simulink model "sampleModel1690_2_sub"  (R2023a)
settings: Solver=VariableStepAuto  StartTime=0.0  StopTime=10.0  RelTol=1e-3
libraries: hdlsllib x1, simulink x1
settings Model: Creator=user1  LastModifiedBy=user1

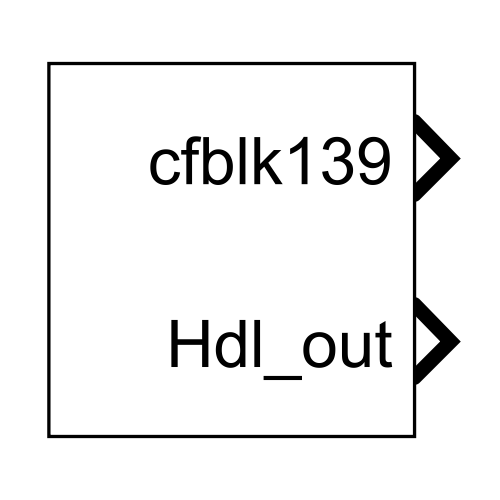
[thumbnail: Simulink's stored preview of the top-level diagram]
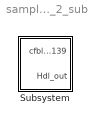
== system sampleModel1690_2_sub ==
  Subsystem : Subsystem

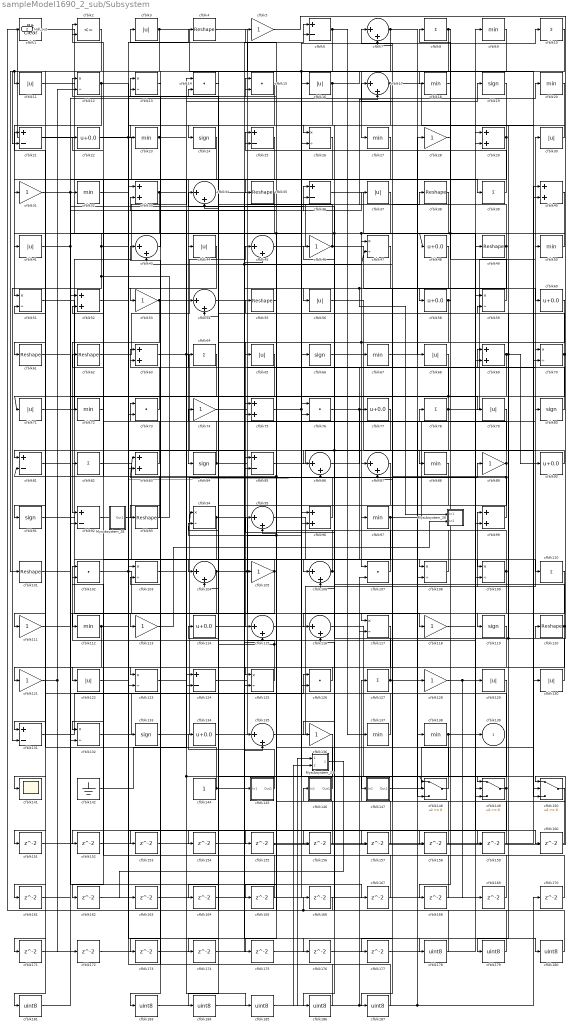
== system sampleModel1690_2_sub/Subsystem ==
  Mysubsystem_23 : Subsystem  TreatAsAtomicUnit=on  RTWFcnName=Mysubsystem_23
      settings: RTWFcnNameOpts=User specified  RTWFileNameOpts=Use function name
  Mysubsystem_26 : Subsystem  TreatAsAtomicUnit=on  RTWFcnName=Mysubsystem_26
      settings: RTWFcnNameOpts=User specified  RTWFileNameOpts=Use function name
  Mysubsystem_28 : Subsystem  TreatAsAtomicUnit=on  RTWFcnName=Mysubsystem_28
      settings: RTWFcnNameOpts=User specified  RTWFileNameOpts=Use function name
  cfblk1 : simulink/Logic and Bit Operations/Bit Clear  iBit=0
      settings: LibrarySourceBlock=|
      | hdlsllib/Logic and Bit
      | Operations/Bit Clear
  cfblk{8,10,39,64,78,82,110,127} (8 alike) : Sum  Inputs=+  OutDataTypeStr=uint8
  cfblk{4,35,38,49,55,61..62,93,101,120} (10 alike) : Reshape
  cfblk{14..15,73,76,102,107,126} (7 alike) : DotProduct  OutDataTypeStr=uint8
  cfblk{12..13,26,47,51,59,70,94,103,108..109,117,123,125,132} (15 alike) : Product  Inputs=*/  OutDataTypeStr=uint8  RndMeth=Zero  SaturateOnIntegerOverflow=on
  cfblk{7,17,34,43,45,54,86..87,95,104,106,115..116,135} (14 alike) : Sum  Inputs=|++  OutDataTypeStr=uint8
  cfblk{5,28,31,46,53,74,89,105,111,113,118,121,128,136} (14 alike) : Gain  OutDataTypeStr=uint8
  cfblk{3,11,16,30,37,41,44,56,65,68,71,79,122,129..130} (15 alike) : Abs  OutDataTypeStr=uint8  SaturateOnIntegerOverflow=off
  cfblk{9,18,20,23,27,32,50,67,72,88,97,112,137..138} (14 alike) : MinMax  OutDataTypeStr=uint8
  cfblk{22,48,58,60,77,90,114,134} (8 alike) : Bias  Bias=0.0  SaturateOnIntegerOverflow=off
  cfblk{19,24,66,80,84,91,119,133} (8 alike) : Signum
  cfblk{6,21,25,36,81,85,92,124,131} (9 alike) : Sum  Inputs=+-  OutDataTypeStr=uint8
  cfblk141 : Scope
  cfblk142 : Ground
  cfblk144 : Constant  OutDataTypeStr=uint8  SampleTime=-1
  cfblk145 : Subsystem
      settings: LibrarySourceBlock=|
      | hdlsllib/Ports &
      | Subsystems/Subsystem
  cfblk146 : Subsystem
      settings: LibrarySourceBlock=|
      | hdlsllib/Ports &
      | Subsystems/Subsystem
  cfblk147 : Subsystem
      settings: LibrarySourceBlock=|
      | hdlsllib/Ports &
      | Subsystems/Subsystem
  cfblk148 : Switch  OutDataTypeStr=uint8  SaturateOnIntegerOverflow=off  InputSameDT=off
  cfblk149 : Switch  OutDataTypeStr=uint8  SaturateOnIntegerOverflow=off  InputSameDT=off
  cfblk150 : Switch  OutDataTypeStr=uint8  SaturateOnIntegerOverflow=off  InputSameDT=off
  cfblk{151..177} (27 alike) : Delay  SampleTime=1
  cfblk{178..181,183..187} (9 alike) : DataTypeConversion  OutDataTypeStr=uint8  SaturateOnIntegerOverflow=off  RndMeth=Floor
  cfblk2 : RelationalOperator  Operator=<=  OutDataTypeStr=boolean  InputSameDT=off
  cfblk{29,33,40,52,63,69,75,83,96,99} (10 alike) : Sum  OutDataTypeStr=uint8
  cfblk139 : Outport  OutDataTypeStr=uint8  VectorParamsAs1DForOutWhenUnconnected=off
  Hdl_out : Outport  Port=2  OutDataTypeStr=uint8
  wires:
  cfblk82/1 -> cfblk106/1
  cfblk115/1 -> cfblk30/1
  cfblk31/1 -> cfblk167/1, cfblk39/1
  cfblk51/1 -> cfblk113/1
  cfblk135/1 -> cfblk99/1
  cfblk78/1 -> cfblk125/2, cfblk50/1, cfblk71/1, cfblk7/2
  cfblk12/1 -> cfblk35/1, cfblk51/1
  cfblk84/1 -> cfblk22/1, cfblk78/1
  cfblk74/1 -> cfblk69/1
  cfblk26/1 -> cfblk84/1
  cfblk15/1 -> cfblk24/1
  cfblk133/1 -> cfblk89/1
  cfblk4/1 -> cfblk27/1
  cfblk2/1 -> cfblk101/1
  cfblk134/1 -> cfblk6/1
  cfblk94/1 -> cfblk112/1, cfblk118/1
  cfblk71/1 -> cfblk14/1
  cfblk96/1 -> cfblk14/2
  cfblk54/1 -> cfblk38/1
  cfblk43/1 -> cfblk13/1
  cfblk37/1 -> cfblk61/1
  cfblk8/1 -> cfblk58/1, cfblk53/1
  cfblk105/1 -> cfblk132/2, cfblk104/1
  cfblk97/1 -> cfblk105/1, cfblk49/1
  cfblk132/1 -> cfblk126/1
  cfblk95/1 -> cfblk109/1
  cfblk121/1 -> cfblk172/1, cfblk12/2
  cfblk27/1 -> cfblk81/1
  cfblk99/1 -> cfblk43/2, cfblk83/1
  cfblk116/1 -> cfblk149/1
  cfblk24/1 -> cfblk31/1
  cfblk144/1 -> cfblk51/2, cfblk6/2, cfblk47/2
  cfblk1/1 -> cfblk76/2
  cfblk30/1 -> cfblk26/1
  cfblk91/1 -> cfblk110/1
  cfblk79/1 -> cfblk116/1
  cfblk53/1 -> cfblk37/1, cfblk92/1
  cfblk123/1 -> cfblk159/1, cfblk148/1
  cfblk64/1 -> cfblk91/1
  cfblk125/1 -> cfblk94/2, cfblk102/1
  cfblk29/1 -> cfblk153/1, cfblk23/1
  cfblk145/1(Out1) -> cfblk134/1
  cfblk102/1 -> cfblk86/2, cfblk145/1(In1)
  cfblk67/1 -> cfblk28/1
  cfblk112/1 -> cfblk161/1, cfblk4/1
  cfblk150/1 -> cfblk127/1
  cfblk17/1 -> cfblk106/2, cfblk40/2
  cfblk14/1 -> cfblk104/2
  cfblk40/1 -> cfblk93/1, cfblk107/1
  cfblk19/1 -> cfblk56/1
  cfblk111/1 -> cfblk72/1
  cfblk101/1 -> cfblk20/1
  cfblk50/1 -> cfblk47/1
  cfblk68/1 -> cfblk92/2
  cfblk90/1 -> cfblk82/1
  cfblk89/1 -> cfblk177/1, cfblk62/1
  cfblk127/1 -> cfblk80/1, cfblk55/1
  cfblk81/1 -> cfblk36/1
  cfblk120/1 -> cfblk148/2, cfblk34/1
  cfblk87/1 -> cfblk97/1
  cfblk3/1 -> cfblk150/2, cfblk21/2, cfblk11/1
  cfblk45/1 -> cfblk17/2
  cfblk106/1 -> cfblk64/1, cfblk46/1
  cfblk63/1 -> cfblk117/1, cfblk115/1
  cfblk41/1 -> cfblk73/2, cfblk44/1
  cfblk70/1 -> cfblk131/1, cfblk13/2
  cfblk11/1 -> cfblk133/1
  cfblk16/1 -> cfblk123/2, cfblk18/1
  cfblk59/1 -> cfblk8/1
  cfblk39/1 -> cfblk25/1
  cfblk85/1 -> cfblk87/1
  cfblk23/1 -> Hdl_out/1, cfblk19/1
  cfblk93/1 -> cfblk2/1
  cfblk75/1 -> cfblk150/3, cfblk10/1
  cfblk33/1 -> cfblk181/1, cfblk176/1
  cfblk80/1 -> cfblk43/1
  cfblk77/1 -> cfblk186/1, cfblk121/1
  cfblk61/1 -> cfblk36/2
  cfblk56/1 -> cfblk130/1
  cfblk114/1 -> cfblk178/1
  cfblk28/1 -> cfblk48/1, cfblk88/1
  cfblk108/1 -> cfblk3/1
  cfblk146/1(Out1) -> cfblk73/1
  cfblk5/1 -> cfblk120/1
  cfblk52/1 -> cfblk79/1
  cfblk69/1 -> cfblk175/1, cfblk90/1, cfblk119/1
  cfblk6/1 -> cfblk151/1, cfblk137/1
  cfblk130/1 -> cfblk59/2, cfblk95/1
  cfblk107/1 -> cfblk33/2
  cfblk110/1 -> cfblk136/1
  cfblk128/1 -> cfblk169/1, cfblk59/1
  cfblk46/1 -> cfblk12/1, cfblk60/1
  cfblk21/1 -> cfblk138/1
  cfblk76/1 -> cfblk108/1, cfblk139/1
  cfblk124/1 -> cfblk9/1
  cfblk55/1 -> cfblk125/1
  cfblk86/1 -> cfblk70/1
  cfblk10/1 -> cfblk141/1
  cfblk72/1 -> cfblk2/2
  cfblk34/1 -> cfblk135/2
  cfblk103/1 -> cfblk185/1
  cfblk47/1 -> cfblk75/2, Mysubsystem_26/1(In1)
  cfblk65/1 -> cfblk111/1
  cfblk36/1 -> cfblk129/1
  cfblk62/1 -> cfblk45/1
  cfblk58/1 -> cfblk168/1, cfblk85/1
  cfblk147/1(Out1) -> cfblk70/2
  cfblk109/1 -> cfblk187/1, cfblk74/1
  cfblk137/1 -> cfblk5/1
  cfblk49/1 -> cfblk147/1(In1), cfblk7/1
  cfblk9/1 -> cfblk123/1, cfblk96/2
  cfblk60/1 -> cfblk174/1, cfblk77/1
  cfblk83/1 -> cfblk52/2
  cfblk138/1 -> cfblk148/3, cfblk29/2
  cfblk149/1 -> cfblk152/1, cfblk21/1
  cfblk7/1 -> cfblk54/2, cfblk68/1
  cfblk22/1 -> cfblk85/2, cfblk124/1
  cfblk38/1 -> cfblk86/1, cfblk65/1, cfblk124/2
  cfblk44/1 -> cfblk83/2
  cfblk126/1 -> cfblk122/1
  cfblk142/1 -> cfblk54/1
  cfblk131/1 -> cfblk66/1
  cfblk148/1 -> cfblk94/1, cfblk25/2, cfblk81/2
  cfblk73/1 -> cfblk63/1
  cfblk104/1 -> cfblk132/1, cfblk16/1, cfblk126/2
  cfblk66/1 -> cfblk67/1
  cfblk151/1 -> cfblk26/2
  cfblk152/1 -> cfblk45/2
  cfblk153/1 -> cfblk40/1
  cfblk119/1 -> cfblk154/1
  cfblk154/1 -> cfblk135/1
  cfblk92/1 -> cfblk155/1
  cfblk155/1 -> cfblk150/1
  cfblk129/1 -> cfblk156/1
  cfblk156/1 -> cfblk95/2
  cfblk122/1 -> cfblk157/1
  cfblk157/1 -> cfblk96/1
  cfblk18/1 -> cfblk158/1
  cfblk158/1 -> cfblk87/2
  cfblk159/1 -> cfblk17/1
  cfblk118/1 -> cfblk160/1
  cfblk160/1 -> cfblk149/2
  cfblk161/1 -> cfblk52/1
  cfblk25/1 -> cfblk162/1
  cfblk162/1 -> cfblk99/2
  cfblk163/1 -> cfblk76/1
  cfblk88/1 -> cfblk164/1
  cfblk164/1 -> cfblk34/2
  cfblk48/1 -> cfblk165/1
  cfblk165/1 -> cfblk102/2
  cfblk166/1 -> cfblk1/1
  cfblk167/1 -> cfblk33/1
  cfblk168/1 -> cfblk75/1
  cfblk169/1 -> cfblk116/2
  cfblk170/1 -> cfblk63/2
  cfblk117/1 -> cfblk171/1
  cfblk171/1 -> cfblk109/2
  cfblk172/1 -> cfblk29/1
  cfblk35/1 -> cfblk173/1
  cfblk173/1 -> cfblk69/2
  cfblk174/1 -> cfblk115/2
  cfblk175/1 -> cfblk149/3
  cfblk176/1 -> cfblk107/2
  cfblk177/1 -> cfblk108/2
  cfblk178/1 -> cfblk15/2, cfblk166/1
  cfblk20/1 -> cfblk179/1
  cfblk179/1 -> cfblk114/1
  cfblk32/1 -> cfblk180/1
  cfblk180/1 -> cfblk146/1(In1)
  cfblk181/1 -> cfblk32/1
  cfblk13/1 -> cfblk183/1
  cfblk136/1 -> cfblk184/1
  cfblk185/1 -> cfblk117/2, cfblk128/1, cfblk170/1
  cfblk186/1 -> cfblk103/1
  cfblk187/1 -> cfblk103/2
  cfblk183/1 -> Mysubsystem_23/1(In1)
  cfblk184/1 -> Mysubsystem_23/2(In2)
  Mysubsystem_23/1(Out1) -> cfblk163/1
  cfblk113/1 -> Mysubsystem_26/2(In2)
  Mysubsystem_28/1(Out1) -> cfblk131/2, cfblk15/1, cfblk41/1

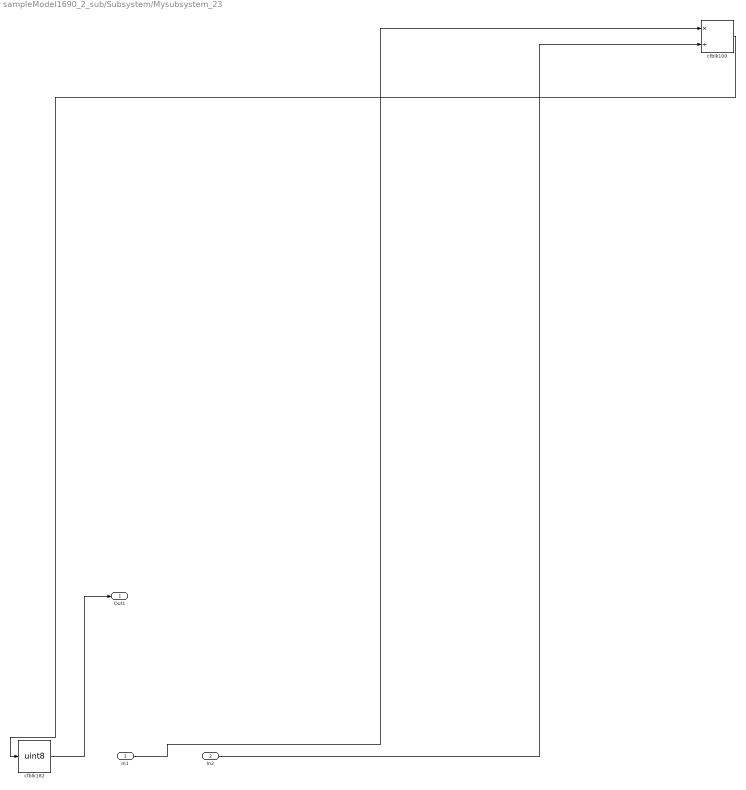
== system sampleModel1690_2_sub/Subsystem/Mysubsystem_23 ==
  In1 : Inport
  In2 : Inport  Port=2
  cfblk100 : Product  Inputs=*/  RndMeth=Zero  SaturateOnIntegerOverflow=on
  cfblk182 : DataTypeConversion  OutDataTypeStr=uint8  SaturateOnIntegerOverflow=off  RndMeth=Floor
  Out1 : Outport
  wires:
  In1/1 -> cfblk100/1
  cfblk182/1 -> Out1/1
  In2/1 -> cfblk100/2
  cfblk100/1 -> cfblk182/1

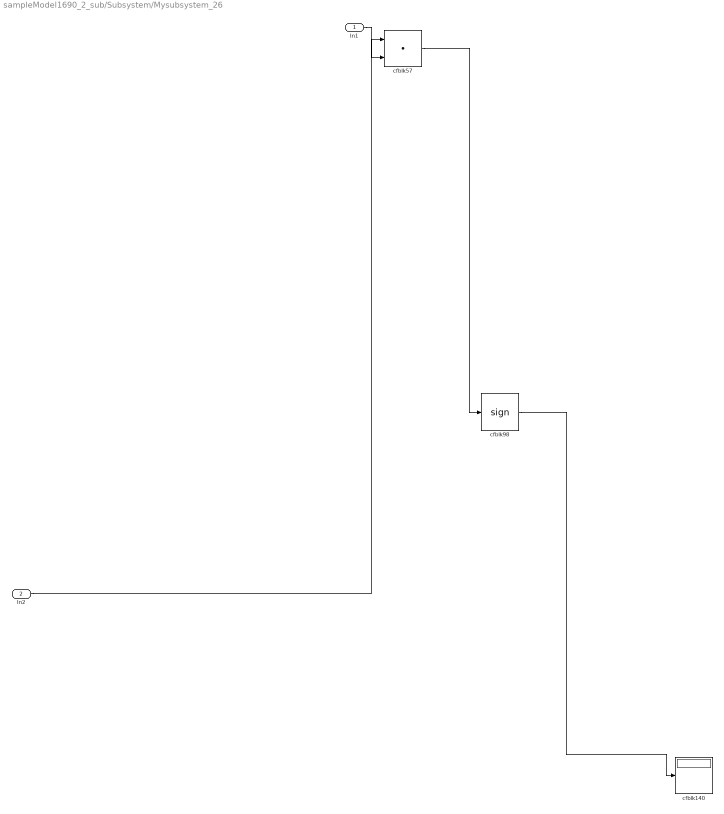
== system sampleModel1690_2_sub/Subsystem/Mysubsystem_26 ==
  In1 : Inport
  In2 : Inport  Port=2
  cfblk140 : Display
  cfblk57 : DotProduct  OutDataTypeStr=Inherit: Inherit via internal rule
  cfblk98 : Signum
  wires:
  In1/1 -> cfblk57/2
  In2/1 -> cfblk57/1
  cfblk98/1 -> cfblk140/1
  cfblk57/1 -> cfblk98/1

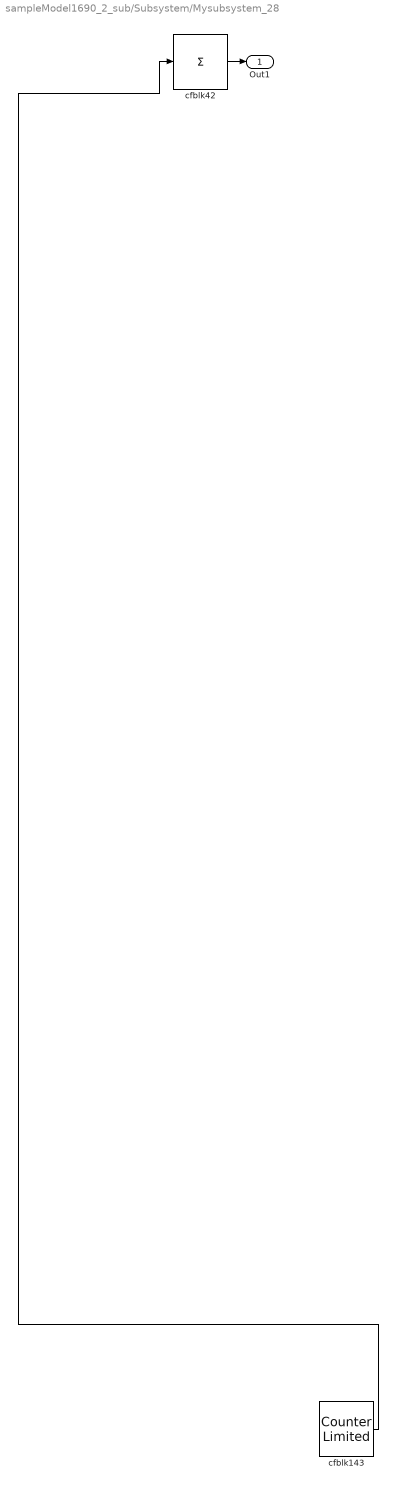
== system sampleModel1690_2_sub/Subsystem/Mysubsystem_28 ==
  cfblk143 : hdlsllib/Sources/Counter Limited  uplimit=7  tsamp=-1
  cfblk42 : Sum  Inputs=+
  Out1 : Outport
  wires:
  cfblk42/1 -> Out1/1
  cfblk143/1 -> cfblk42/1

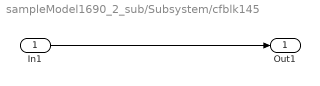
== system sampleModel1690_2_sub/Subsystem/cfblk145 ==
  In1 : Inport
  Out1 : Outport
  wires:
  In1/1 -> Out1/1

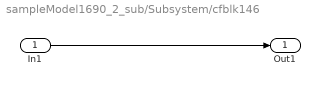
== system sampleModel1690_2_sub/Subsystem/cfblk146 ==
  In1 : Inport
  Out1 : Outport
  wires:
  In1/1 -> Out1/1

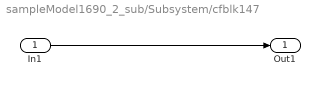
== system sampleModel1690_2_sub/Subsystem/cfblk147 ==
  In1 : Inport
  Out1 : Outport
  wires:
  In1/1 -> Out1/1
